simulink model "sldemo_foreach_repeat_scalar"  (Simulink 7.6)
settings: Solver=FixedStepDiscrete  StartTime=0.0  StopTime=1.0  RelTol=1e-3
settings Model: Creator=The MathWorks Inc.
settings DataIOCC: SaveFormat=Structure
settings OptimizationCC: OptimizeModelRefInitCode=on  LifeSpan=1
settings RTWCC: SystemTargetFile=ert.tlc  TemplateMakefile=ert_default_tmf  Description=Real-Time Workshop Embedded Coder  GenerateReport=on  ProcessScript=ert_make_rtw_hook  IncludeHyperlinkInReport=on  LaunchReport=on
settings CodeAppCC: IgnoreCustomStorageClasses=off
settings ERTTargetCC: MultiwordLength=2048  GenerateSampleERTMain=on  MatFileLogging=on  SupportVariableSizeSignals=on  ERTCustomFileTemplate=example_file_process.tlc  ConvertIfToSwitch=off

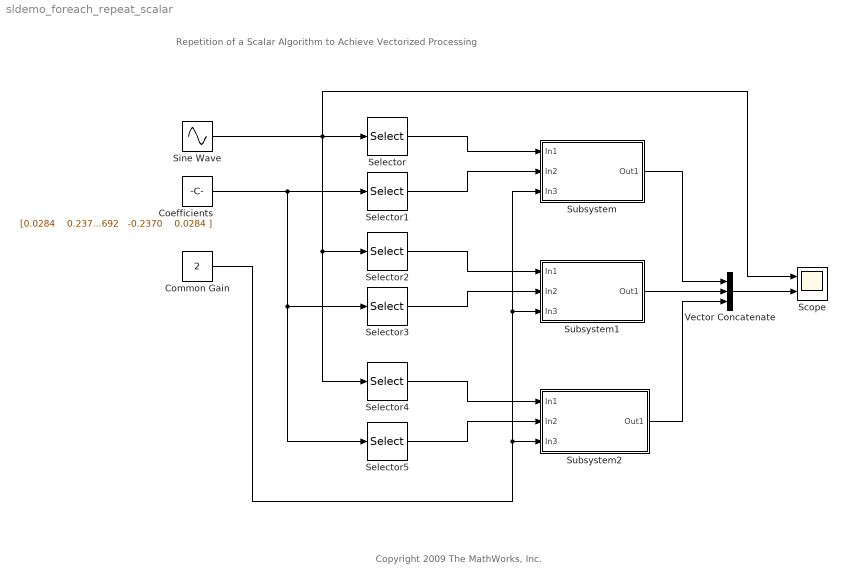
== system sldemo_foreach_repeat_scalar ==
  note: Copyright 2009 The MathWorks, Inc.
  note: Repetition of a Scalar Algorithm to
      | Achieve Vectorized Processing
  Coefficients : Constant  Value=|
      | [0.0284    0.2370    0.4692    0.2370    0.0284
      | ;   -0.0651   -0.0000    0.8698   -0.0000   -0.0651
      |  ;   0.0284   -0.2370    0.4692   -0.2370    0.0284
      | ]
  Common Gain : Constant  Value=2
  Scope : Scope  NumInputPorts=2
      settings: YMin=-5~-5  YMax=5~5
  Selector : Selector  InputPortWidth=3  IndexOptions=Index vector (dialog)  Indices=1  OutputSizes=1
  Selector1 : Selector  NumberOfDimensions=2  InputPortWidth=3  IndexOptions=Index vector (dialog),Select all  Indices=1,1  OutputSizes=1,1
  Selector2 : Selector  InputPortWidth=3  IndexOptions=Index vector (dialog)  Indices=2  OutputSizes=1
  Selector3 : Selector  NumberOfDimensions=2  InputPortWidth=3  IndexOptions=Index vector (dialog),Select all  Indices=2,1  OutputSizes=1,1
  Selector4 : Selector  InputPortWidth=3  IndexOptions=Index vector (dialog)  Indices=3  OutputSizes=1
  Selector5 : Selector  NumberOfDimensions=2  InputPortWidth=3  IndexOptions=Index vector (dialog),Select all  Indices=3,1  OutputSizes=1,1
  Sine Wave : Sin  Amplitude=[1 1 1]  Frequency=[25 15 5]*pi  SampleTime=1/30
  Subsystem : Subsystem
  Subsystem1 : Subsystem
  Subsystem2 : Subsystem
  Vector Concatenate : Concatenate  NumInputs=3  Mode=Vector
  wires:
  Sine Wave/1 -> Selector/1, Selector2/1, Selector4/1, Scope/1
  Subsystem/1(Out1) -> Vector Concatenate/1
  Coefficients/1 -> Selector1/1, Selector3/1, Selector5/1
  Selector1/1 -> Subsystem/2(In2)
  Selector2/1 -> Subsystem1/1(In1)
  Selector3/1 -> Subsystem1/2(In2)
  Selector4/1 -> Subsystem2/1(In1)
  Selector5/1 -> Subsystem2/2(In2)
  Common Gain/1 -> Subsystem2/3(In3), Subsystem/3(In3), Subsystem1/3(In3)
  Subsystem1/1(Out1) -> Vector Concatenate/2
  Subsystem2/1(Out1) -> Vector Concatenate/3
  Vector Concatenate/1 -> Scope/2
  Selector/1 -> Subsystem/1(In1)

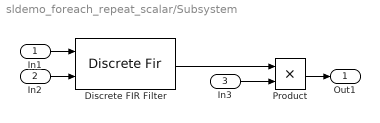
== system sldemo_foreach_repeat_scalar/Subsystem ==
  In1 : Inport
  In2 : Inport  Port=2
  In3 : Inport  Port=3
  Discrete FIR Filter : DiscreteFir  CoefSource=Input port
  Product : Product  RndMeth=Zero
  Out1 : Outport
  wires:
  Discrete FIR Filter/1 -> Product/1
  In3/1 -> Product/2
  In1/1 -> Discrete FIR Filter/1
  In2/1 -> Discrete FIR Filter/2
  Product/1 -> Out1/1

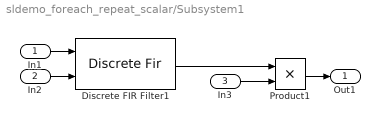
== system sldemo_foreach_repeat_scalar/Subsystem1 ==
  In1 : Inport
  In2 : Inport  Port=2
  In3 : Inport  Port=3
  Discrete FIR Filter1 : DiscreteFir  CoefSource=Input port
  Product1 : Product  RndMeth=Zero
  Out1 : Outport
  wires:
  Discrete FIR Filter1/1 -> Product1/1
  In3/1 -> Product1/2
  In1/1 -> Discrete FIR Filter1/1
  In2/1 -> Discrete FIR Filter1/2
  Product1/1 -> Out1/1

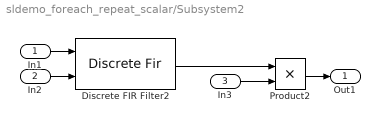
== system sldemo_foreach_repeat_scalar/Subsystem2 ==
  In1 : Inport
  In2 : Inport  Port=2
  In3 : Inport  Port=3
  Discrete FIR Filter2 : DiscreteFir  CoefSource=Input port
  Product2 : Product  RndMeth=Zero
  Out1 : Outport
  wires:
  Discrete FIR Filter2/1 -> Product2/1
  In3/1 -> Product2/2
  In1/1 -> Discrete FIR Filter2/1
  In2/1 -> Discrete FIR Filter2/2
  Product2/1 -> Out1/1
